simulink model "t_t_200_tge5"  (Simulink 6.2)
settings: Solver=ode45  StartTime=0.0  StopTime=10  RelTol=1e-3
undefined symbols (not defined in the file): BEE2_usr
libraries: xbsIndex_r3 x575, xps_library x48, casper_library x20
(part 3 of 4)

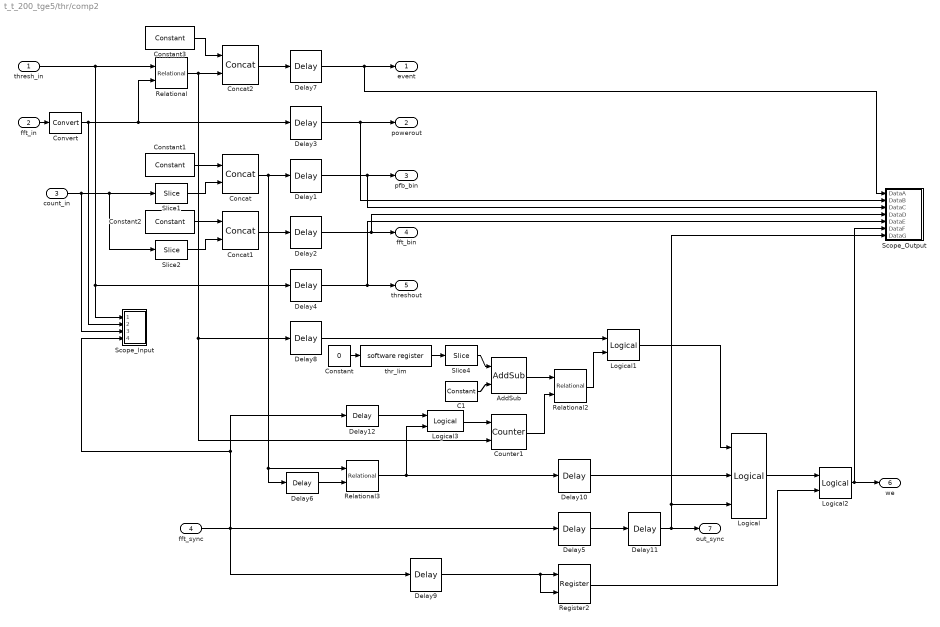
== system t_t_200_tge5/thr/comp2 ==
  thresh_in : Inport  Port=1  LatchInput=off
  fft_in : Inport  Port=2  LatchInput=off
  count_in : Inport  Port=3  LatchInput=off
  fft_sync : Inport  Port=4  LatchInput=off
  AddSub : xbsIndex_r3/AddSub  mode=Subtraction  precision=Full  arith_type=Unsigned  n_bits=8  bin_pt=2  quantization=Truncate  overflow=Wrap  latency=1  explicit_period=off  period=1  use_carryin=off  use_carryout=off  en=off  dbl_ovrd=off  show_param=off  use_core=on  pipeline=off  use_rpm=on  gen_core=off
      settings: xl_area=[0, 0, 0, 0, 0, 0, 0]
  C1 : xbsIndex_r3/Constant  const=1  equ=P=C  arith_type=Unsigned  n_bits=FFTSize  bin_pt=0  opselect=C  inp2=PCIN>>17  opr=+  inp1=P  carry=CIN  iostate=0  explicit_period=on  period=1  dbl_ovrd=off
  Concat : xbsIndex_r3/Concat  num_inputs=2  explicit_period=off  period=1  dbl_ovrd=off
  Concat1 : xbsIndex_r3/Concat  num_inputs=2  explicit_period=off  period=1  dbl_ovrd=off
  Concat2 : xbsIndex_r3/Concat  num_inputs=2  explicit_period=off  period=1  dbl_ovrd=off
  Constant : Constant  Value=0  OutDataTypeMode=double
  Constant1 : xbsIndex_r3/Constant  const=0  equ=P=C  arith_type=Unsigned  n_bits=CPUWidth - PFBSize  bin_pt=0  opselect=C  inp2=PCIN>>17  opr=+  inp1=P  carry=CIN  iostate=0  explicit_period=on  period=1  dbl_ovrd=off
  Constant2 : xbsIndex_r3/Constant  const=0  equ=P=C  arith_type=Unsigned  n_bits=CPUWidth - FFTSize  bin_pt=0  opselect=C  inp2=PCIN>>17  opr=+  inp1=P  carry=CIN  iostate=0  explicit_period=on  period=1  dbl_ovrd=off
  Constant3 : xbsIndex_r3/Constant  const=0  equ=P=C  arith_type=Unsigned  n_bits=CPUWidth-1  bin_pt=0  opselect=C  inp2=PCIN>>17  opr=+  inp1=P  carry=CIN  iostate=0  explicit_period=on  period=1  dbl_ovrd=off
  Convert : xbsIndex_r3/Convert  arith_type=Unsigned  n_bits=CPUWidth  bin_pt=CPUWidth - 3  quantization=Truncate  overflow=Wrap  latency=0  explicit_period=off  period=1  dbl_ovrd=off  show_param=off  inserted_by_tool=off  pipeline=off
      settings: xl_area=[0, 0, 0, 0, 0, 0, 0]
  Counter1 : xbsIndex_r3/Counter  cnt_type=Free Running  n_bits=FFTSize  bin_pt=0  arith_type=Unsigned  start_count=0  cnt_to=Inf  cnt_by_val=1  operation=Up  explicit_period=off  period=1  load_pin=off  rst=on  en=on  dbl_ovrd=off  show_param=off  use_rpm=on  gen_core=off
      settings: xl_area=[0, 0, 0, 0, 0, 0, 0]
  Delay{1..4} (4 alike) : xbsIndex_r3/Delay  latency=3  reg_retiming=on  explicit_period=off  period=1  en=off  accept_only_valid=off  init_zero=on  dbl_ovrd=off  show_param=off
      settings: xl_area=[0, 0, 0, 0, 0, 0, 0]
  Delay{6,8,10..12} (5 alike) : xbsIndex_r3/Delay  latency=1  reg_retiming=on  explicit_period=off  period=1  en=off  accept_only_valid=off  init_zero=on  dbl_ovrd=off  show_param=off
      settings: xl_area=[0, 0, 0, 0, 0, 0, 0]
  Delay5 : xbsIndex_r3/Delay  latency=2  reg_retiming=on  explicit_period=off  period=1  en=off  accept_only_valid=off  init_zero=on  dbl_ovrd=off  show_param=off
      settings: xl_area=[0, 0, 0, 0, 0, 0, 0]
  Delay7 : xbsIndex_r3/Delay  latency=2  reg_retiming=on  explicit_period=off  period=1  en=off  accept_only_valid=off  init_zero=on  dbl_ovrd=off  show_param=off
      settings: xl_area=[0, 0, 0, 0, 0, 0, 0]
  Delay9 : xbsIndex_r3/Delay  latency=2  reg_retiming=on  explicit_period=off  period=1  en=off  accept_only_valid=off  init_zero=on  dbl_ovrd=off  show_param=off
      settings: xl_area=[0, 0, 0, 0, 0, 0, 0]
  Logical : xbsIndex_r3/Logical  logical_function=OR  inputs=3  precision=Full  arith_type=Unsigned  n_bits=8  bin_pt=2  align_bp=on  latency=0  explicit_period=off  period=1  en=off  dbl_ovrd=off  show_param=off
      settings: xl_area=[0, 0, 0, 0, 0, 0, 0]
  Logical1 : xbsIndex_r3/Logical  logical_function=AND  inputs=2  precision=Full  arith_type=Unsigned  n_bits=8  bin_pt=2  align_bp=on  latency=0  explicit_period=off  period=1  en=off  dbl_ovrd=off  show_param=off
      settings: xl_area=[0, 0, 0, 0, 0, 0, 0]
  Logical2 : xbsIndex_r3/Logical  logical_function=AND  inputs=2  precision=Full  arith_type=Unsigned  n_bits=8  bin_pt=2  align_bp=on  latency=1  explicit_period=off  period=1  en=off  dbl_ovrd=off  show_param=off
      settings: xl_area=[0, 0, 0, 0, 0, 0, 0]
  Logical3 : xbsIndex_r3/Logical  logical_function=OR  inputs=2  precision=Full  arith_type=Unsigned  n_bits=8  bin_pt=2  align_bp=on  latency=0  explicit_period=off  period=1  en=off  dbl_ovrd=off  show_param=off
      settings: xl_area=[0, 0, 0, 0, 0, 0, 0]
  Register2 : xbsIndex_r3/Register  init=0  reg_only_valid=off  explicit_period=off  period=1  rst=off  en=on  out_en=off  dbl_ovrd=off  show_param=off
      settings: xl_area=[0, 0, 0, 0, 0, 0, 0]
  Relational : xbsIndex_r3/Relational  mode=a<b  latency=1  explicit_period=off  period=1  en=off  dbl_ovrd=off  show_param=off
      settings: xl_area=[0, 0, 0, 0, 0, 0, 0]
  Relational2 : xbsIndex_r3/Relational  mode=a>b  latency=1  explicit_period=off  period=1  en=off  dbl_ovrd=off  show_param=off
      settings: xl_area=[0, 0, 0, 0, 0, 0, 0]
  Relational3 : xbsIndex_r3/Relational  mode=a!=b  latency=1  explicit_period=off  period=1  en=off  dbl_ovrd=off  show_param=off
      settings: xl_area=[0, 0, 0, 0, 0, 0, 0]
  Scope_Input : Subsystem
  Scope_Output : Subsystem
  Slice1 : xbsIndex_r3/Slice  mode=Lower Bit Location + Width  nbits=PFBSize  bit1=0  base1=MSB of Input  bit0=FFTSize  base0=LSB of Input  boolean_output=off  explicit_period=off  period=1  dbl_ovrd=off
  Slice2 : xbsIndex_r3/Slice  mode=Lower Bit Location + Width  nbits=FFTSize  bit1=0  base1=MSB of Input  bit0=0  base0=LSB of Input  boolean_output=off  explicit_period=off  period=1  dbl_ovrd=off
  Slice4 : xbsIndex_r3/Slice  mode=Lower Bit Location + Width  nbits=FFTSize  bit1=0  base1=MSB of Input  bit0=0  base0=LSB of Input  boolean_output=off  explicit_period=off  period=1  dbl_ovrd=off
  thr_lim : xps_library/software register  Tag=xps:sw_reg  io_dir=From Processor  arith_type=Unsigned  bitwidth=32  bin_pt=0  sample_period=1  gw_name=t_t_200_tge5_thr_comp2_thr_lim_user_data_out
  event : Outport
  powerout : Outport  Port=2
  pfb_bin : Outport  Port=3
  fft_bin : Outport  Port=4
  threshout : Outport  Port=5
  we : Outport  Port=6
  out_sync : Outport  Port=7
  wires:
  thresh_in/1 -> Relational/1, Scope_Input/1(DataA), Delay4/1
  Relational/1 -> Delay8/1, Counter1/2, Concat2/2
  fft_in/1 -> Convert/1
  Delay3/1 -> powerout/1, Scope_Output/2(DataB)
  Slice2/1 -> Concat1/2
  Constant2/1 -> Concat1/1
  Slice1/1 -> Concat/2
  Constant1/1 -> Concat/1
  count_in/1 -> Slice1/1, Slice2/1, Scope_Input/3(DataC)
  Concat/1 -> Delay1/1, Relational3/1, Delay6/1
  Concat1/1 -> Delay2/1
  Delay1/1 -> pfb_bin/1, Scope_Output/3(DataC)
  Delay2/1 -> fft_bin/1, Scope_Output/4(DataD)
  Delay4/1 -> Scope_Output/5(DataE), threshout/1
  fft_sync/1 -> Scope_Input/4(Sync), Delay12/1, Delay5/1, Delay9/1
  Delay5/1 -> Delay11/1
  Constant/1 -> thr_lim/1
  thr_lim/1 -> Slice4/1
  Relational3/1 -> Delay10/1, Logical3/2
  Delay6/1 -> Relational3/2
  Relational2/1 -> Logical1/2
  Logical1/1 -> Logical/1
  Delay7/1 -> event/1, Scope_Output/1(DataA)
  Delay8/1 -> Logical1/1
  Slice4/1 -> AddSub/1
  C1/1 -> AddSub/2
  Counter1/1 -> Relational2/2
  AddSub/1 -> Relational2/1
  Delay10/1 -> Logical/2
  Concat2/1 -> Delay7/1
  Constant3/1 -> Concat2/1
  Logical3/1 -> Counter1/1
  Delay11/1 -> Scope_Output/7("DataG "), Logical/3, out_sync/1
  Logical/1 -> Logical2/1
  Logical2/1 -> we/1, Scope_Output/6("DataF ")
  Delay9/1 -> Register2/1, Register2/2
  Delay12/1 -> Logical3/1
  Register2/1 -> Logical2/2
  Convert/1 -> Delay3/1, Relational/2, Scope_Input/2(DataB)

== system t_t_200_tge5/thr/ct_power ==
  note: Reloaded 'c_to_ri' blocks.
      | May need to change
      | bitwidth and binary point
  din1 : Inport  Port=1  LatchInput=off
  din2 : Inport  Port=2  LatchInput=off
  din_sync : Inport  Port=3  LatchInput=off
  Scope_Input : Subsystem
  a1 : xbsIndex_r3/AddSub  mode=Addition  precision=Full  arith_type=Unsigned  n_bits=8  bin_pt=2  quantization=Truncate  overflow=Wrap  latency=add_lat  explicit_period=off  period=1  use_carryin=off  use_carryout=off  en=off  dbl_ovrd=off  show_param=off  use_core=on  pipeline=off  use_rpm=on  gen_core=off
      settings: xl_area=[0, 0, 0, 0, 0, 0, 0]
  a2 : xbsIndex_r3/AddSub  mode=Addition  precision=Full  arith_type=Unsigned  n_bits=8  bin_pt=2  quantization=Truncate  overflow=Wrap  latency=add_lat  explicit_period=off  period=1  use_carryin=off  use_carryout=off  en=off  dbl_ovrd=off  show_param=off  use_core=on  pipeline=off  use_rpm=on  gen_core=off
      settings: xl_area=[0, 0, 0, 0, 0, 0, 0]
  c_to_ri : casper_library/Misc/c_to_ri  n_bits=DataWidth  bin_pt=DataWidth - 1
      settings: AttributesFormatString=18_17 r/i
  c_to_ri1 : casper_library/Misc/c_to_ri  n_bits=DataWidth  bin_pt=DataWidth -1
      settings: AttributesFormatString=18_17 r/i
  delay_sync : xbsIndex_r3/Delay  latency=add_lat+mult_lat  reg_retiming=off  explicit_period=off  period=1  en=off  accept_only_valid=off  init_zero=on  dbl_ovrd=off  show_param=off
      settings: xl_area=[0, 0, 0, 0, 0, 0, 0]
  m{1..4} (4 alike) : xbsIndex_r3/Mult  precision=Full  arith_type=Unsigned  n_bits=2*DataWidth  bin_pt=2*(DataWidth-1)  quantization="Round  (unbiased: +/- Inf)"  overflow=Wrap  latency=mult_lat  explicit_period=on  period=-1  en=off  dbl_ovrd=off  show_param=on  mult_type=Parallel  oversample=2  use_embedded=on  pipeline=on  use_rpm=on  placement_style=Rectangular Shape  gen_core=off
      settings: xl_area=[0, 0, 0, 0, 0, 0, 0]
  pout1 : Outport
  pout2 : Outport  Port=2
  dout_sync : Outport  Port=3
  wires:
  din1/1 -> c_to_ri/1
  c_to_ri/1 -> Scope_Input/1(DataA), m1/1, m1/2
  c_to_ri/2 -> m2/2, m2/1, Scope_Input/2(DataB)
  din2/1 -> c_to_ri1/1
  c_to_ri1/1 -> m3/2, m3/1
  m2/1 -> Scope_Input/3(DataC), a1/2
  a1/1 -> Scope_Input/4(Sync), pout1/1
  m3/1 -> a2/1
  m4/1 -> a2/2
  a2/1 -> pout2/1
  m1/1 -> a1/1
  c_to_ri1/2 -> m4/1, m4/2
  delay_sync/1 -> dout_sync/1
  din_sync/1 -> delay_sync/1

== system t_t_200_tge5/thr/fft_power ==
  note: Reloaded 'c_to_ri' blocks.
      | May need to change
      | bitwidth and binary point
  din1 : Inport  Port=1  LatchInput=off
  din2 : Inport  Port=2  LatchInput=off
  din_sync : Inport  Port=3  LatchInput=off
  Scope_Input : Subsystem
  a1 : xbsIndex_r3/AddSub  mode=Addition  precision=Full  arith_type=Unsigned  n_bits=8  bin_pt=2  quantization=Truncate  overflow=Wrap  latency=add_lat  explicit_period=off  period=1  use_carryin=off  use_carryout=off  en=off  dbl_ovrd=off  show_param=off  use_core=on  pipeline=off  use_rpm=on  gen_core=off
      settings: xl_area=[0, 0, 0, 0, 0, 0, 0]
  a2 : xbsIndex_r3/AddSub  mode=Addition  precision=Full  arith_type=Unsigned  n_bits=8  bin_pt=2  quantization=Truncate  overflow=Wrap  latency=add_lat  explicit_period=off  period=1  use_carryin=off  use_carryout=off  en=off  dbl_ovrd=off  show_param=off  use_core=on  pipeline=off  use_rpm=on  gen_core=off
      settings: xl_area=[0, 0, 0, 0, 0, 0, 0]
  c_to_ri : casper_library/Misc/c_to_ri  n_bits=DataWidth  bin_pt=DataWidth-1
      settings: AttributesFormatString=18_17 r/i
  c_to_ri1 : casper_library/Misc/c_to_ri  n_bits=DataWidth  bin_pt=DataWidth - 1
      settings: AttributesFormatString=18_17 r/i
  delay_sync : xbsIndex_r3/Delay  latency=add_lat+mult_lat  reg_retiming=off  explicit_period=off  period=1  en=off  accept_only_valid=off  init_zero=on  dbl_ovrd=off  show_param=off
      settings: xl_area=[0, 0, 0, 0, 0, 0, 0]
  m{1..4} (4 alike) : xbsIndex_r3/Mult  precision=User Defined  arith_type=Unsigned  n_bits=2*DataWidth  bin_pt=2*(DataWidth-1)  quantization="Round  (unbiased: +/- Inf)"  overflow=Wrap  latency=mult_lat  explicit_period=on  period=-1  en=off  dbl_ovrd=off  show_param=on  mult_type=Parallel  oversample=2  use_embedded=on  pipeline=on  use_rpm=on  placement_style=Rectangular Shape  gen_core=off
      settings: xl_area=[0, 0, 0, 0, 0, 0, 0]
  pout1 : Outport
  pout2 : Outport  Port=2
  dout_sync : Outport  Port=3
  wires:
  din1/1 -> Scope_Input/3(DataC), c_to_ri/1
  c_to_ri/1 -> m1/1, m1/2
  c_to_ri/2 -> m2/1, m2/2
  din2/1 -> c_to_ri1/1
  c_to_ri1/1 -> m3/1, m3/2
  m2/1 -> a1/2
  a1/1 -> Scope_Input/1(DataA), pout1/1
  m3/1 -> a2/1
  m4/1 -> a2/2
  a2/1 -> Scope_Input/2(DataB), pout2/1
  m1/1 -> a1/1
  c_to_ri1/2 -> m4/2, m4/1
  delay_sync/1 -> Scope_Input/4(Sync), dout_sync/1
  din_sync/1 -> delay_sync/1

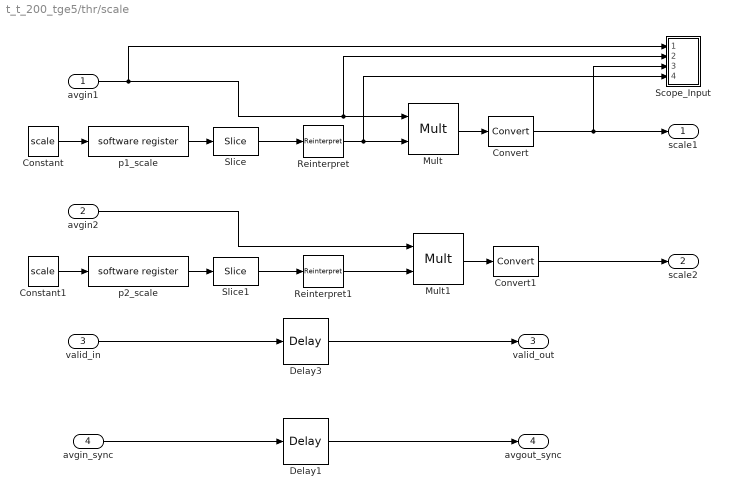
== system t_t_200_tge5/thr/scale ==
  avgin1 : Inport  Port=1  LatchInput=off
  avgin2 : Inport  Port=2  LatchInput=off
  valid_in : Inport  Port=3  LatchInput=off
  avgin_sync : Inport  Port=4  LatchInput=off
  Constant : Constant  Value=scale
  Constant1 : Constant  Value=scale
  Convert : xbsIndex_r3/Convert  arith_type=Unsigned  n_bits=2*DataWidth  bin_pt=2*DataWidth-2  quantization=Truncate  overflow=Wrap  latency=0  explicit_period=off  period=1  dbl_ovrd=off  show_param=off  inserted_by_tool=off  pipeline=off
      settings: xl_area=[0, 0, 0, 0, 0, 0, 0]
  Convert1 : xbsIndex_r3/Convert  arith_type=Unsigned  n_bits=2*DataWidth  bin_pt=2*DataWidth-2  quantization=Truncate  overflow=Wrap  latency=0  explicit_period=off  period=1  dbl_ovrd=off  show_param=off  inserted_by_tool=off  pipeline=off
      settings: xl_area=[0, 0, 0, 0, 0, 0, 0]
  Delay1 : xbsIndex_r3/Delay  latency=3  reg_retiming=off  explicit_period=off  period=1  en=off  accept_only_valid=off  init_zero=on  dbl_ovrd=off  show_param=off
      settings: xl_area=[0, 0, 0, 0, 0, 0, 0]
  Delay3 : xbsIndex_r3/Delay  latency=3  reg_retiming=off  explicit_period=off  period=1  en=off  accept_only_valid=off  init_zero=on  dbl_ovrd=off  show_param=off
      settings: xl_area=[0, 0, 0, 0, 0, 0, 0]
  Mult : xbsIndex_r3/Mult  precision=Full  arith_type="Signed  (2's comp)"  n_bits=8  bin_pt=2  quantization=Truncate  overflow=Wrap  latency=mult_lat  explicit_period=off  period=1  en=off  dbl_ovrd=off  show_param=on  mult_type=Parallel  oversample=2  use_embedded=on  pipeline=on  use_rpm=on  placement_style=Rectangular Shape  gen_core=off
      settings: xl_area=[0, 0, 0, 0, 0, 0, 0]
  Mult1 : xbsIndex_r3/Mult  precision=Full  arith_type="Signed  (2's comp)"  n_bits=8  bin_pt=2  quantization=Truncate  overflow=Wrap  latency=mult_lat  explicit_period=off  period=1  en=off  dbl_ovrd=off  show_param=on  mult_type=Parallel  oversample=2  use_embedded=on  pipeline=on  use_rpm=on  placement_style=Rectangular Shape  gen_core=off
      settings: xl_area=[0, 0, 0, 0, 0, 0, 0]
  Reinterpret : xbsIndex_r3/Reinterpret  force_arith_type=on  arith_type=Unsigned  force_bin_pt=on  bin_pt=DataWidth - ceil(DataWidth/2)  force_valid=on
  Reinterpret1 : xbsIndex_r3/Reinterpret  force_arith_type=on  arith_type=Unsigned  force_bin_pt=on  bin_pt=DataWidth - ceil(DataWidth/2)  force_valid=on
  Scope_Input : Subsystem
  Slice : xbsIndex_r3/Slice  mode=Lower Bit Location + Width  nbits=DataWidth  bit1=0  base1=LSB of Input  bit0=0  base0=LSB of Input  boolean_output=off  explicit_period=off  period=1  dbl_ovrd=off
  Slice1 : xbsIndex_r3/Slice  mode=Lower Bit Location + Width  nbits=DataWidth  bit1=0  base1=LSB of Input  bit0=0  base0=LSB of Input  boolean_output=off  explicit_period=off  period=1  dbl_ovrd=off
  p1_scale : xps_library/software register  Tag=xps:sw_reg  io_dir=From Processor  arith_type=Unsigned  bitwidth=32  bin_pt=ceil(DataWidth/2)  sample_period=1  gw_name=t_t_200_tge5_thr_scale_p1_scale_user_data_out
  p2_scale : xps_library/software register  Tag=xps:sw_reg  io_dir=From Processor  arith_type=Unsigned  bitwidth=32  bin_pt=ceil(DataWidth/2)  sample_period=1  gw_name=t_t_200_tge5_thr_scale_p2_scale_user_data_out
  scale1 : Outport
  scale2 : Outport  Port=2
  valid_out : Outport  Port=3
  avgout_sync : Outport  Port=4
  wires:
  Convert1/1 -> scale2/1
  Convert/1 -> Scope_Input/3(DataC), scale1/1
  avgin_sync/1 -> Delay1/1
  Delay1/1 -> avgout_sync/1
  Constant1/1 -> p2_scale/1
  Constant/1 -> p1_scale/1
  avgin2/1 -> Mult1/1
  Slice/1 -> Reinterpret/1
  Slice1/1 -> Reinterpret1/1
  p1_scale/1 -> Slice/1
  p2_scale/1 -> Slice1/1
  Reinterpret/1 -> Scope_Input/4(Sync), Mult/2
  avgin1/1 -> Scope_Input/2(DataB), Mult/1, Scope_Input/1(DataA)
  Reinterpret1/1 -> Mult1/2
  Mult/1 -> Convert/1
  Mult1/1 -> Convert1/1
  valid_in/1 -> Delay3/1
  Delay3/1 -> valid_out/1

== system t_t_200_tge5/ct_in_mux/tvg/bram_wr_out_sim ==
  Concat : xbsIndex_r3/Concat  num_inputs=5  explicit_period=off  period=1  dbl_ovrd=off
  Gateway Out : xbsIndex_r3/Gateway Out  output_type=Double  nbits=8  bin_pt=6  arith_type=Boolean  quantization=Truncate  overflow=Wrap  hdl_port=on  timing_constraint=None  locs_specified=off  LOCs={}  needs_fixed_name=off  show_param=off
      settings: xl_area=[0, 0, 0, 0, 0, 0, 0]
  RAM_sel : xbsIndex_r3/Constant  const=ram_sel  equ=P=C  arith_type=Unsigned  n_bits=2  bin_pt=0  opselect=C  inp2=PCIN>>17  opr=+  inp1=P  carry=CIN  iostate=0  explicit_period=on  period=1  dbl_ovrd=off
  WE : xbsIndex_r3/Constant  const=we_enable  equ=P=C  arith_type=Unsigned  n_bits=1  bin_pt=0  opselect=C  inp2=PCIN>>17  opr=+  inp1=P  carry=CIN  iostate=0  explicit_period=on  period=1  dbl_ovrd=off
  add_vec : xbsIndex_r3/Constant  const=add_vec  equ=P=C  arith_type=Unsigned  n_bits=9  bin_pt=0  opselect=C  inp2=PCIN>>17  opr=+  inp1=P  carry=CIN  iostate=0  explicit_period=on  period=1  dbl_ovrd=off
  data_in : xbsIndex_r3/Constant  const=data_in  equ=P=C  arith_type=Unsigned  n_bits=18  bin_pt=0  opselect=C  inp2=PCIN>>17  opr=+  inp1=P  carry=CIN  iostate=0  explicit_period=on  period=1  dbl_ovrd=off
  zeros : xbsIndex_r3/Constant  const=0  equ=P=C  arith_type=Unsigned  n_bits=2  bin_pt=0  opselect=C  inp2=PCIN>>17  opr=+  inp1=P  carry=CIN  iostate=0  explicit_period=on  period=1  dbl_ovrd=off
  Out1 : Outport
  wires:
  Gateway Out/1 -> Out1/1
  Concat/1 -> Gateway Out/1
  zeros/1 -> Concat/1
  WE/1 -> Concat/2
  RAM_sel/1 -> Concat/3
  add_vec/1 -> Concat/4
  data_in/1 -> Concat/5

== system t_t_200_tge5/ct_in_mux/tvg/thr_cpu_ctrl_sim ==
  Concat : xbsIndex_r3/Concat  num_inputs=4  explicit_period=off  period=1  dbl_ovrd=off
  Delay : xbsIndex_r3/Delay  latency=1  reg_retiming=off  explicit_period=off  period=1  en=off  accept_only_valid=off  init_zero=on  dbl_ovrd=off  show_param=off
      settings: xl_area=[0, 0, 0, 0, 0, 0, 0]
  Disregard Subsystem : xbsIndex_r3/Disregard Subsystem  Tag=discardX
      settings: AttributesFormatString=Disregard Subsystem\nFor Generation
  Gateway Out : xbsIndex_r3/Gateway Out  output_type=Double  nbits=8  bin_pt=6  arith_type=Boolean  quantization=Truncate  overflow=Wrap  hdl_port=off  timing_constraint=None  locs_specified=off  LOCs={}  needs_fixed_name=off  show_param=off
      settings: xl_area=[0, 0, 0, 0, 0, 0, 0]
  Length : xbsIndex_r3/Constant  const=tvg_length  equ=P=C  arith_type=Unsigned  n_bits=10  bin_pt=0  opselect=C  inp2=PCIN>>17  opr=+  inp1=P  carry=CIN  iostate=0  explicit_period=on  period=1  dbl_ovrd=off
  "Skip\t" : xbsIndex_r3/Constant  const=tvg_skip  equ=P=C  arith_type=Unsigned  n_bits=10  bin_pt=0  opselect=C  inp2=PCIN>>17  opr=+  inp1=P  carry=CIN  iostate=0  explicit_period=on  period=1  dbl_ovrd=off
  Stall : xbsIndex_r3/Constant  const=tvg_stall  equ=P=C  arith_type=Unsigned  n_bits=10  bin_pt=0  opselect=C  inp2=PCIN>>17  opr=+  inp1=P  carry=CIN  iostate=0  explicit_period=on  period=1  dbl_ovrd=off
  pad_zeroes : xbsIndex_r3/Constant  const=0  equ=P=C  arith_type=Unsigned  n_bits=2  bin_pt=0  opselect=C  inp2=PCIN>>17  opr=+  inp1=P  carry=CIN  iostate=0  explicit_period=on  period=1  dbl_ovrd=off
  out : Outport
  wires:
  "Skip\t"/1 -> Concat/4
  Delay/1 -> Gateway Out/1
  Concat/1 -> Delay/1
  Gateway Out/1 -> out/1
  Stall/1 -> Concat/3
  pad_zeroes/1 -> Concat/1
  Length/1 -> Concat/2

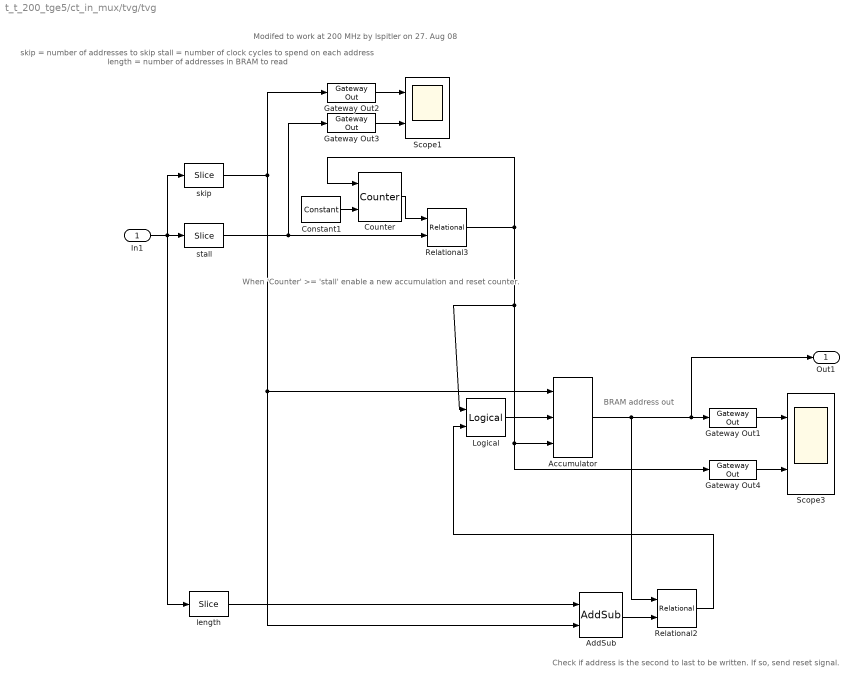
== system t_t_200_tge5/ct_in_mux/tvg/tvg ==
  note: Modifed to work at 200 MHz
      | by lspitler on 27. Aug 08
  note: BRAM address out
  note: Check if address is the
      | second to last to be written.
      | If so, send reset signal.
  note: When 'Counter' >= 'stall'
      | enable a new accumulation
      | and reset counter.
  note: skip = number of addresses to skip
      | stall = number of clock cycles to spend
      | on each address
      | length = number of addresses in BRAM
      | to read
  In1 : Inport  Port=1  LatchInput=off
  Accumulator : xbsIndex_r3/Accumulator  n_bits=10  overflow=Wrap  operation=Add  scale=1  explicit_period=on  period=1  rst=on  hasbypass=off  en=on  dbl_ovrd=off  show_param=off  gen_core=off  use_rpm=on
      settings: xl_area=[0, 0, 0, 0, 0, 0, 0]
  AddSub : xbsIndex_r3/AddSub  mode=Subtraction  precision=Full  arith_type=Unsigned  n_bits=8  bin_pt=2  quantization=Truncate  overflow=Wrap  latency=1  explicit_period=on  period=1  use_carryin=off  use_carryout=off  en=off  dbl_ovrd=off  show_param=off  use_core=on  pipeline=off  use_rpm=on  gen_core=off
      settings: xl_area=[0, 0, 0, 0, 0, 0, 0]
  Constant1 : xbsIndex_r3/Constant  const=1  equ=P=C  arith_type=Unsigned  n_bits=10  bin_pt=0  opselect=C  inp2=PCIN>>17  opr=+  inp1=P  carry=CIN  iostate=0  explicit_period=on  period=1  dbl_ovrd=off
  Counter : xbsIndex_r3/Counter  cnt_type=Free Running  n_bits=10  bin_pt=0  arith_type=Unsigned  start_count=0  cnt_to=inf  cnt_by_val=1  operation=Up  explicit_period=on  period=1  load_pin=on  rst=off  en=off  dbl_ovrd=off  show_param=off  use_rpm=on  gen_core=off
      settings: xl_area=[0, 0, 0, 0, 0, 0, 0]
  Gateway Out{1..4} (4 alike) : xbsIndex_r3/Gateway Out  output_type=Double  nbits=8  bin_pt=6  arith_type=Boolean  quantization=Truncate  overflow=Wrap  hdl_port=on  timing_constraint=None  locs_specified=off  LOCs={}  needs_fixed_name=off  show_param=off
      settings: xl_area=[0, 0, 0, 0, 0, 0, 0]
  Logical : xbsIndex_r3/Logical  logical_function=AND  inputs=2  precision=Full  arith_type=Unsigned  n_bits=8  bin_pt=2  align_bp=on  latency=0  explicit_period=off  period=1  en=off  dbl_ovrd=off  show_param=off
      settings: xl_area=[0, 0, 0, 0, 0, 0, 0]
  Relational2 : xbsIndex_r3/Relational  mode=a>=b  latency=0  explicit_period=on  period=1  en=off  dbl_ovrd=off  show_param=off
      settings: xl_area=[0, 0, 0, 0, 0, 0, 0]
  Relational3 : xbsIndex_r3/Relational  mode=a>=b  latency=0  explicit_period=on  period=1  en=off  dbl_ovrd=off  show_param=off
      settings: xl_area=[0, 0, 0, 0, 0, 0, 0]
  Scope1 : Scope  NumInputPorts=2
      settings: YMin=-5~-5  YMax=5~5
  Scope3 : Scope  NumInputPorts=2
      settings: TimeRange=20  YMin=-5~-5  YMax=5~5  SaveName=ScopeData4
  length : xbsIndex_r3/Slice  mode=Lower Bit Location + Width  nbits=10  bit1=0  base1=MSB of Input  bit0=20  base0=LSB of Input  boolean_output=off  explicit_period=on  period=1  dbl_ovrd=off
  skip : xbsIndex_r3/Slice  mode=Lower Bit Location + Width  nbits=10  bit1=0  base1=MSB of Input  bit0=0  base0=LSB of Input  boolean_output=off  explicit_period=on  period=1  dbl_ovrd=off
  stall : xbsIndex_r3/Slice  mode=Lower Bit Location + Width  nbits=10  bit1=0  base1=MSB of Input  bit0=10  base0=LSB of Input  boolean_output=off  explicit_period=on  period=1  dbl_ovrd=off
  Out1 : Outport
  wires:
  length/1 -> AddSub/1
  AddSub/1 -> Relational2/2
  In1/1 -> stall/1, skip/1, length/1
  Gateway Out1/1 -> Scope3/1
  Accumulator/1 -> Relational2/1, Out1/1, Gateway Out1/1
  skip/1 -> AddSub/2, Accumulator/1, Gateway Out2/1
  stall/1 -> Gateway Out3/1, Relational3/2
  Gateway Out2/1 -> Scope1/1
  Gateway Out3/1 -> Scope1/2
  Gateway Out4/1 -> Scope3/2
  Relational3/1 -> Counter/1, Accumulator/3, Gateway Out4/1, Logical/1
  Counter/1 -> Relational3/1
  Constant1/1 -> Counter/2
  Relational2/1 -> Logical/2
  Logical/1 -> Accumulator/2

== system t_t_200_tge5/fft_in_mux/tvg/bram_wr_out_sim ==
  Concat : xbsIndex_r3/Concat  num_inputs=5  explicit_period=off  period=1  dbl_ovrd=off
  Gateway Out : xbsIndex_r3/Gateway Out  output_type=Double  nbits=8  bin_pt=6  arith_type=Boolean  quantization=Truncate  overflow=Wrap  hdl_port=on  timing_constraint=None  locs_specified=off  LOCs={}  needs_fixed_name=off  show_param=off
      settings: xl_area=[0, 0, 0, 0, 0, 0, 0]
  RAM_sel : xbsIndex_r3/Constant  const=ram_sel  equ=P=C  arith_type=Unsigned  n_bits=2  bin_pt=0  opselect=C  inp2=PCIN>>17  opr=+  inp1=P  carry=CIN  iostate=0  explicit_period=on  period=1  dbl_ovrd=off
  WE : xbsIndex_r3/Constant  const=we_enable  equ=P=C  arith_type=Unsigned  n_bits=1  bin_pt=0  opselect=C  inp2=PCIN>>17  opr=+  inp1=P  carry=CIN  iostate=0  explicit_period=on  period=1  dbl_ovrd=off
  add_vec : xbsIndex_r3/Constant  const=add_vec  equ=P=C  arith_type=Unsigned  n_bits=9  bin_pt=0  opselect=C  inp2=PCIN>>17  opr=+  inp1=P  carry=CIN  iostate=0  explicit_period=on  period=1  dbl_ovrd=off
  data_in : xbsIndex_r3/Constant  const=data_in  equ=P=C  arith_type=Unsigned  n_bits=18  bin_pt=0  opselect=C  inp2=PCIN>>17  opr=+  inp1=P  carry=CIN  iostate=0  explicit_period=on  period=1  dbl_ovrd=off
  zeros : xbsIndex_r3/Constant  const=0  equ=P=C  arith_type=Unsigned  n_bits=2  bin_pt=0  opselect=C  inp2=PCIN>>17  opr=+  inp1=P  carry=CIN  iostate=0  explicit_period=on  period=1  dbl_ovrd=off
  Out1 : Outport
  wires:
  Gateway Out/1 -> Out1/1
  Concat/1 -> Gateway Out/1
  zeros/1 -> Concat/1
  WE/1 -> Concat/2
  RAM_sel/1 -> Concat/3
  add_vec/1 -> Concat/4
  data_in/1 -> Concat/5

== system t_t_200_tge5/fft_in_mux/tvg/thr_cpu_ctrl_sim ==
  Concat : xbsIndex_r3/Concat  num_inputs=4  explicit_period=off  period=1  dbl_ovrd=off
  Delay : xbsIndex_r3/Delay  latency=1  reg_retiming=off  explicit_period=off  period=1  en=off  accept_only_valid=off  init_zero=on  dbl_ovrd=off  show_param=off
      settings: xl_area=[0, 0, 0, 0, 0, 0, 0]
  Disregard Subsystem : xbsIndex_r3/Disregard Subsystem  Tag=discardX
      settings: AttributesFormatString=Disregard Subsystem\nFor Generation
  Gateway Out : xbsIndex_r3/Gateway Out  output_type=Double  nbits=8  bin_pt=6  arith_type=Boolean  quantization=Truncate  overflow=Wrap  hdl_port=off  timing_constraint=None  locs_specified=off  LOCs={}  needs_fixed_name=off  show_param=off
      settings: xl_area=[0, 0, 0, 0, 0, 0, 0]
  Length : xbsIndex_r3/Constant  const=tvg_length  equ=P=C  arith_type=Unsigned  n_bits=10  bin_pt=0  opselect=C  inp2=PCIN>>17  opr=+  inp1=P  carry=CIN  iostate=0  explicit_period=on  period=1  dbl_ovrd=off
  "Skip\t" : xbsIndex_r3/Constant  const=tvg_skip  equ=P=C  arith_type=Unsigned  n_bits=10  bin_pt=0  opselect=C  inp2=PCIN>>17  opr=+  inp1=P  carry=CIN  iostate=0  explicit_period=on  period=1  dbl_ovrd=off
  Stall : xbsIndex_r3/Constant  const=tvg_stall  equ=P=C  arith_type=Unsigned  n_bits=10  bin_pt=0  opselect=C  inp2=PCIN>>17  opr=+  inp1=P  carry=CIN  iostate=0  explicit_period=on  period=1  dbl_ovrd=off
  pad_zeroes : xbsIndex_r3/Constant  const=0  equ=P=C  arith_type=Unsigned  n_bits=2  bin_pt=0  opselect=C  inp2=PCIN>>17  opr=+  inp1=P  carry=CIN  iostate=0  explicit_period=on  period=1  dbl_ovrd=off
  out : Outport
  wires:
  "Skip\t"/1 -> Concat/4
  Delay/1 -> Gateway Out/1
  Concat/1 -> Delay/1
  Gateway Out/1 -> out/1
  Stall/1 -> Concat/3
  pad_zeroes/1 -> Concat/1
  Length/1 -> Concat/2

== system t_t_200_tge5/fft_in_mux/tvg/tvg ==
  note: Modifed to work at 200 MHz
      | by lspitler on 27. Aug 08
  note: BRAM address out
  note: Check if address is the
      | second to last to be written.
      | If so, send reset signal.
  note: When 'Counter' >= 'stall'
      | enable a new accumulation
      | and reset counter.
  note: skip = number of addresses to skip
      | stall = number of clock cycles to spend
      | on each address
      | length = number of addresses in BRAM
      | to read
  In1 : Inport  Port=1  LatchInput=off
  Accumulator : xbsIndex_r3/Accumulator  n_bits=10  overflow=Wrap  operation=Add  scale=1  explicit_period=on  period=1  rst=on  hasbypass=off  en=on  dbl_ovrd=off  show_param=off  gen_core=off  use_rpm=on
      settings: xl_area=[0, 0, 0, 0, 0, 0, 0]
  AddSub : xbsIndex_r3/AddSub  mode=Subtraction  precision=Full  arith_type=Unsigned  n_bits=8  bin_pt=2  quantization=Truncate  overflow=Wrap  latency=1  explicit_period=on  period=1  use_carryin=off  use_carryout=off  en=off  dbl_ovrd=off  show_param=off  use_core=on  pipeline=off  use_rpm=on  gen_core=off
      settings: xl_area=[0, 0, 0, 0, 0, 0, 0]
  Constant1 : xbsIndex_r3/Constant  const=1  equ=P=C  arith_type=Unsigned  n_bits=10  bin_pt=0  opselect=C  inp2=PCIN>>17  opr=+  inp1=P  carry=CIN  iostate=0  explicit_period=on  period=1  dbl_ovrd=off
  Counter : xbsIndex_r3/Counter  cnt_type=Free Running  n_bits=10  bin_pt=0  arith_type=Unsigned  start_count=0  cnt_to=inf  cnt_by_val=1  operation=Up  explicit_period=on  period=1  load_pin=on  rst=off  en=off  dbl_ovrd=off  show_param=off  use_rpm=on  gen_core=off
      settings: xl_area=[0, 0, 0, 0, 0, 0, 0]
  Gateway Out{1..4} (4 alike) : xbsIndex_r3/Gateway Out  output_type=Double  nbits=8  bin_pt=6  arith_type=Boolean  quantization=Truncate  overflow=Wrap  hdl_port=on  timing_constraint=None  locs_specified=off  LOCs={}  needs_fixed_name=off  show_param=off
      settings: xl_area=[0, 0, 0, 0, 0, 0, 0]
  Logical : xbsIndex_r3/Logical  logical_function=AND  inputs=2  precision=Full  arith_type=Unsigned  n_bits=8  bin_pt=2  align_bp=on  latency=0  explicit_period=off  period=1  en=off  dbl_ovrd=off  show_param=off
      settings: xl_area=[0, 0, 0, 0, 0, 0, 0]
  Relational2 : xbsIndex_r3/Relational  mode=a>=b  latency=0  explicit_period=on  period=1  en=off  dbl_ovrd=off  show_param=off
      settings: xl_area=[0, 0, 0, 0, 0, 0, 0]
  Relational3 : xbsIndex_r3/Relational  mode=a>=b  latency=0  explicit_period=on  period=1  en=off  dbl_ovrd=off  show_param=off
      settings: xl_area=[0, 0, 0, 0, 0, 0, 0]
  Scope1 : Scope  NumInputPorts=2
      settings: YMin=-5~-5  YMax=5~5
  Scope3 : Scope  NumInputPorts=2
      settings: TimeRange=20  YMin=-5~-5  YMax=5~5  SaveName=ScopeData4
  length : xbsIndex_r3/Slice  mode=Lower Bit Location + Width  nbits=10  bit1=0  base1=MSB of Input  bit0=20  base0=LSB of Input  boolean_output=off  explicit_period=on  period=1  dbl_ovrd=off
  skip : xbsIndex_r3/Slice  mode=Lower Bit Location + Width  nbits=10  bit1=0  base1=MSB of Input  bit0=0  base0=LSB of Input  boolean_output=off  explicit_period=on  period=1  dbl_ovrd=off
  stall : xbsIndex_r3/Slice  mode=Lower Bit Location + Width  nbits=10  bit1=0  base1=MSB of Input  bit0=10  base0=LSB of Input  boolean_output=off  explicit_period=on  period=1  dbl_ovrd=off
  Out1 : Outport
  wires:
  length/1 -> AddSub/1
  AddSub/1 -> Relational2/2
  In1/1 -> stall/1, skip/1, length/1
  Gateway Out1/1 -> Scope3/1
  Accumulator/1 -> Relational2/1, Out1/1, Gateway Out1/1
  skip/1 -> AddSub/2, Accumulator/1, Gateway Out2/1
  stall/1 -> Gateway Out3/1, Relational3/2
  Gateway Out2/1 -> Scope1/1
  Gateway Out3/1 -> Scope1/2
  Gateway Out4/1 -> Scope3/2
  Relational3/1 -> Counter/1, Accumulator/3, Gateway Out4/1, Logical/1
  Counter/1 -> Relational3/1
  Constant1/1 -> Counter/2
  Relational2/1 -> Logical/2
  Logical/1 -> Accumulator/2

== system t_t_200_tge5/thr/avg/Scope_Input ==
  DataA : Inport  Port=1  LatchInput=off
  DataB : Inport  Port=2  LatchInput=off
  DataC : Inport  Port=3  LatchInput=off
  Sync : Inport  Port=4  LatchInput=off
  Gateway Out{1..4} (4 alike) : xbsIndex_r3/Gateway Out  output_type=Double  nbits=8  bin_pt=6  arith_type=Boolean  quantization=Truncate  overflow=Wrap  hdl_port=off  timing_constraint=None  locs_specified=off  LOCs={}  needs_fixed_name=off  show_param=off
      settings: xl_area=[0, 0, 0, 0, 0, 0, 0]
  scope_ct_p1 : Scope  NumInputPorts=4
      settings: TimeRange=225.9933774834437  YMin=0~0~0~0  YMax=0.014~0.02~140~1
  wires:
  Sync/1 -> Gateway Out4/1
  Gateway Out4/1 -> scope_ct_p1/4
  DataC/1 -> Gateway Out3/1
  Gateway Out3/1 -> scope_ct_p1/3
  DataA/1 -> Gateway Out2/1
  Gateway Out1/1 -> scope_ct_p1/2
  DataB/1 -> Gateway Out1/1
  Gateway Out2/1 -> scope_ct_p1/1

== system t_t_200_tge5/thr/comp1/in_fft ==
  din : Inport  Port=1  LatchInput=off
  trig : Inport  Port=2  LatchInput=off
  en : Inport  Port=3  LatchInput=off
  Constant5 : xbsIndex_r3/Constant  const=1  equ=P=C  arith_type=Boolean  n_bits=1  bin_pt=0  opselect=C  inp2=PCIN>>17  opr=+  inp1=P  carry=CIN  iostate=0  explicit_period=on  period=1  dbl_ovrd=off
  Gateway Out : xbsIndex_r3/Gateway Out  output_type=Double  nbits=8  bin_pt=6  arith_type=Boolean  quantization=Truncate  overflow=Wrap  hdl_port=off  timing_constraint=None  locs_specified=off  LOCs={}  needs_fixed_name=off  show_param=off
      settings: xl_area=[0, 0, 0, 0, 0, 0, 0]
  Gateway Out1 : xbsIndex_r3/Gateway Out  output_type=Double  nbits=8  bin_pt=6  arith_type=Boolean  quantization=Truncate  overflow=Wrap  hdl_port=off  timing_constraint=None  locs_specified=off  LOCs={}  needs_fixed_name=off  show_param=off
      settings: xl_area=[0, 0, 0, 0, 0, 0, 0]
  Logical : xbsIndex_r3/Logical  logical_function=AND  inputs=2  precision=Full  arith_type=Unsigned  n_bits=8  bin_pt=2  align_bp=on  latency=0  explicit_period=on  period=1  en=off  dbl_ovrd=off  show_param=off
      settings: xl_area=[0, 0, 0, 0, 0, 0, 0]
  Reinterpret : xbsIndex_r3/Reinterpret  force_arith_type=on  arith_type=Unsigned  force_bin_pt=on  bin_pt=0  force_valid=on
  Scope : Scope  NumInputPorts=2
      settings: YMin=-5~-5  YMax=5~5
  bram : xps_library/Shared BRAM  Tag=xps:bram  arith_type=Unsigned  addr_width=nsamples  data_width=32  data_bin_pt=0  init_vals=zeros(1,4096)  sample_rate=1
  freeze_cntr : Subsystem  mask{CounterBits=nsamples}
      mask prompts: CounterBits "Counter Length (2^?)"
  posedge : Subsystem  Tag=Rising Edge Detector
  wires:
  Gateway Out1/1 -> Scope/2
  Gateway Out/1 -> Scope/1
  bram/1 -> Gateway Out/1
  freeze_cntr/1(addr) -> bram/1
  en/1 -> Logical/1
  trig/1 -> Logical/2
  posedge/1(Out) -> freeze_cntr/2(rst)
  Logical/1 -> posedge/1(In)
  freeze_cntr/2(we) -> Gateway Out1/1, bram/3
  Constant5/1 -> freeze_cntr/1(en)
  Reinterpret/1 -> bram/2
  din/1 -> Reinterpret/1

== system t_t_200_tge5/thr/comp1/in_thr ==
  din : Inport  Port=1  LatchInput=off
  trig : Inport  Port=2  LatchInput=off
  en : Inport  Port=3  LatchInput=off
  Constant5 : xbsIndex_r3/Constant  const=1  equ=P=C  arith_type=Boolean  n_bits=1  bin_pt=0  opselect=C  inp2=PCIN>>17  opr=+  inp1=P  carry=CIN  iostate=0  explicit_period=on  period=1  dbl_ovrd=off
  Gateway Out : xbsIndex_r3/Gateway Out  output_type=Double  nbits=8  bin_pt=6  arith_type=Boolean  quantization=Truncate  overflow=Wrap  hdl_port=off  timing_constraint=None  locs_specified=off  LOCs={}  needs_fixed_name=off  show_param=off
      settings: xl_area=[0, 0, 0, 0, 0, 0, 0]
  Gateway Out1 : xbsIndex_r3/Gateway Out  output_type=Double  nbits=8  bin_pt=6  arith_type=Boolean  quantization=Truncate  overflow=Wrap  hdl_port=off  timing_constraint=None  locs_specified=off  LOCs={}  needs_fixed_name=off  show_param=off
      settings: xl_area=[0, 0, 0, 0, 0, 0, 0]
  Logical : xbsIndex_r3/Logical  logical_function=AND  inputs=2  precision=Full  arith_type=Unsigned  n_bits=8  bin_pt=2  align_bp=on  latency=0  explicit_period=on  period=1  en=off  dbl_ovrd=off  show_param=off
      settings: xl_area=[0, 0, 0, 0, 0, 0, 0]
  Reinterpret : xbsIndex_r3/Reinterpret  force_arith_type=on  arith_type=Unsigned  force_bin_pt=on  bin_pt=0  force_valid=on
  Scope : Scope  NumInputPorts=2
      settings: YMin=-5~-5  YMax=5~5
  bram : xps_library/Shared BRAM  Tag=xps:bram  arith_type=Unsigned  addr_width=nsamples  data_width=32  data_bin_pt=0  init_vals=zeros(1,4096)  sample_rate=1
  freeze_cntr : Subsystem  mask{CounterBits=nsamples}
      mask prompts: CounterBits "Counter Length (2^?)"
  posedge : Subsystem  Tag=Rising Edge Detector
  wires:
  din/1 -> Reinterpret/1
  Reinterpret/1 -> bram/2
  Constant5/1 -> freeze_cntr/1(en)
  freeze_cntr/2(we) -> bram/3, Gateway Out1/1
  Logical/1 -> posedge/1(In)
  posedge/1(Out) -> freeze_cntr/2(rst)
  trig/1 -> Logical/2
  en/1 -> Logical/1
  freeze_cntr/1(addr) -> bram/1
  bram/1 -> Gateway Out/1
  Gateway Out/1 -> Scope/1
  Gateway Out1/1 -> Scope/2

== system t_t_200_tge5/thr/comp1/out_event ==
  din : Inport  Port=1  LatchInput=off
  trig : Inport  Port=2  LatchInput=off
  en : Inport  Port=3  LatchInput=off
  Constant5 : xbsIndex_r3/Constant  const=1  equ=P=C  arith_type=Boolean  n_bits=1  bin_pt=0  opselect=C  inp2=PCIN>>17  opr=+  inp1=P  carry=CIN  iostate=0  explicit_period=on  period=1  dbl_ovrd=off
  Gateway Out : xbsIndex_r3/Gateway Out  output_type=Double  nbits=8  bin_pt=6  arith_type=Boolean  quantization=Truncate  overflow=Wrap  hdl_port=off  timing_constraint=None  locs_specified=off  LOCs={}  needs_fixed_name=off  show_param=off
      settings: xl_area=[0, 0, 0, 0, 0, 0, 0]
  Gateway Out1 : xbsIndex_r3/Gateway Out  output_type=Double  nbits=8  bin_pt=6  arith_type=Boolean  quantization=Truncate  overflow=Wrap  hdl_port=off  timing_constraint=None  locs_specified=off  LOCs={}  needs_fixed_name=off  show_param=off
      settings: xl_area=[0, 0, 0, 0, 0, 0, 0]
  Logical : xbsIndex_r3/Logical  logical_function=AND  inputs=2  precision=Full  arith_type=Unsigned  n_bits=8  bin_pt=2  align_bp=on  latency=0  explicit_period=on  period=1  en=off  dbl_ovrd=off  show_param=off
      settings: xl_area=[0, 0, 0, 0, 0, 0, 0]
  Reinterpret : xbsIndex_r3/Reinterpret  force_arith_type=on  arith_type=Unsigned  force_bin_pt=on  bin_pt=0  force_valid=on
  Scope : Scope  NumInputPorts=2
      settings: YMin=-5~-5  YMax=5~5
  bram : xps_library/Shared BRAM  Tag=xps:bram  arith_type=Unsigned  addr_width=nsamples  data_width=32  data_bin_pt=0  init_vals=zeros(1,4096)  sample_rate=1
  freeze_cntr : Subsystem  mask{CounterBits=nsamples}
      mask prompts: CounterBits "Counter Length (2^?)"
  posedge : Subsystem  Tag=Rising Edge Detector
  wires:
  din/1 -> Reinterpret/1
  Reinterpret/1 -> bram/2
  Constant5/1 -> freeze_cntr/1(en)
  freeze_cntr/2(we) -> bram/3, Gateway Out1/1
  Logical/1 -> posedge/1(In)
  posedge/1(Out) -> freeze_cntr/2(rst)
  trig/1 -> Logical/2
  en/1 -> Logical/1
  freeze_cntr/1(addr) -> bram/1
  bram/1 -> Gateway Out/1
  Gateway Out/1 -> Scope/1
  Gateway Out1/1 -> Scope/2

== system t_t_200_tge5/thr/comp1/out_fft ==
  din : Inport  Port=1  LatchInput=off
  trig : Inport  Port=2  LatchInput=off
  en : Inport  Port=3  LatchInput=off
  Constant5 : xbsIndex_r3/Constant  const=1  equ=P=C  arith_type=Boolean  n_bits=1  bin_pt=0  opselect=C  inp2=PCIN>>17  opr=+  inp1=P  carry=CIN  iostate=0  explicit_period=on  period=1  dbl_ovrd=off
  Gateway Out : xbsIndex_r3/Gateway Out  output_type=Double  nbits=8  bin_pt=6  arith_type=Boolean  quantization=Truncate  overflow=Wrap  hdl_port=off  timing_constraint=None  locs_specified=off  LOCs={}  needs_fixed_name=off  show_param=off
      settings: xl_area=[0, 0, 0, 0, 0, 0, 0]
  Gateway Out1 : xbsIndex_r3/Gateway Out  output_type=Double  nbits=8  bin_pt=6  arith_type=Boolean  quantization=Truncate  overflow=Wrap  hdl_port=off  timing_constraint=None  locs_specified=off  LOCs={}  needs_fixed_name=off  show_param=off
      settings: xl_area=[0, 0, 0, 0, 0, 0, 0]
  Logical : xbsIndex_r3/Logical  logical_function=AND  inputs=2  precision=Full  arith_type=Unsigned  n_bits=8  bin_pt=2  align_bp=on  latency=0  explicit_period=on  period=1  en=off  dbl_ovrd=off  show_param=off
      settings: xl_area=[0, 0, 0, 0, 0, 0, 0]
  Reinterpret : xbsIndex_r3/Reinterpret  force_arith_type=on  arith_type=Unsigned  force_bin_pt=on  bin_pt=0  force_valid=on
  Scope : Scope  NumInputPorts=2
      settings: YMin=-5~-5  YMax=5~5
  bram : xps_library/Shared BRAM  Tag=xps:bram  arith_type=Unsigned  addr_width=nsamples  data_width=32  data_bin_pt=0  init_vals=zeros(1,4096)  sample_rate=1
  freeze_cntr : Subsystem  mask{CounterBits=nsamples}
      mask prompts: CounterBits "Counter Length (2^?)"
  posedge : Subsystem  Tag=Rising Edge Detector
  wires:
  Gateway Out1/1 -> Scope/2
  Gateway Out/1 -> Scope/1
  bram/1 -> Gateway Out/1
  freeze_cntr/1(addr) -> bram/1
  en/1 -> Logical/1
  trig/1 -> Logical/2
  posedge/1(Out) -> freeze_cntr/2(rst)
  Logical/1 -> posedge/1(In)
  freeze_cntr/2(we) -> Gateway Out1/1, bram/3
  Constant5/1 -> freeze_cntr/1(en)
  Reinterpret/1 -> bram/2
  din/1 -> Reinterpret/1

== system t_t_200_tge5/thr/comp1/out_pfb ==
  din : Inport  Port=1  LatchInput=off
  trig : Inport  Port=2  LatchInput=off
  en : Inport  Port=3  LatchInput=off
  Constant5 : xbsIndex_r3/Constant  const=1  equ=P=C  arith_type=Boolean  n_bits=1  bin_pt=0  opselect=C  inp2=PCIN>>17  opr=+  inp1=P  carry=CIN  iostate=0  explicit_period=on  period=1  dbl_ovrd=off
  Gateway Out : xbsIndex_r3/Gateway Out  output_type=Double  nbits=8  bin_pt=6  arith_type=Boolean  quantization=Truncate  overflow=Wrap  hdl_port=off  timing_constraint=None  locs_specified=off  LOCs={}  needs_fixed_name=off  show_param=off
      settings: xl_area=[0, 0, 0, 0, 0, 0, 0]
  Gateway Out1 : xbsIndex_r3/Gateway Out  output_type=Double  nbits=8  bin_pt=6  arith_type=Boolean  quantization=Truncate  overflow=Wrap  hdl_port=off  timing_constraint=None  locs_specified=off  LOCs={}  needs_fixed_name=off  show_param=off
      settings: xl_area=[0, 0, 0, 0, 0, 0, 0]
  Logical : xbsIndex_r3/Logical  logical_function=AND  inputs=2  precision=Full  arith_type=Unsigned  n_bits=8  bin_pt=2  align_bp=on  latency=0  explicit_period=on  period=1  en=off  dbl_ovrd=off  show_param=off
      settings: xl_area=[0, 0, 0, 0, 0, 0, 0]
  Reinterpret : xbsIndex_r3/Reinterpret  force_arith_type=on  arith_type=Unsigned  force_bin_pt=on  bin_pt=0  force_valid=on
  Scope : Scope  NumInputPorts=2
      settings: YMin=-5~-5  YMax=5~5
  bram : xps_library/Shared BRAM  Tag=xps:bram  arith_type=Unsigned  addr_width=nsamples  data_width=32  data_bin_pt=0  init_vals=zeros(1,4096)  sample_rate=1
  freeze_cntr : Subsystem  mask{CounterBits=nsamples}
      mask prompts: CounterBits "Counter Length (2^?)"
  posedge : Subsystem  Tag=Rising Edge Detector
  wires:
  din/1 -> Reinterpret/1
  Reinterpret/1 -> bram/2
  Constant5/1 -> freeze_cntr/1(en)
  freeze_cntr/2(we) -> bram/3, Gateway Out1/1
  Logical/1 -> posedge/1(In)
  posedge/1(Out) -> freeze_cntr/2(rst)
  trig/1 -> Logical/2
  en/1 -> Logical/1
  freeze_cntr/1(addr) -> bram/1
  bram/1 -> Gateway Out/1
  Gateway Out/1 -> Scope/1
  Gateway Out1/1 -> Scope/2

== system t_t_200_tge5/thr/comp1/out_pwr ==
  din : Inport  Port=1  LatchInput=off
  trig : Inport  Port=2  LatchInput=off
  en : Inport  Port=3  LatchInput=off
  Constant5 : xbsIndex_r3/Constant  const=1  equ=P=C  arith_type=Boolean  n_bits=1  bin_pt=0  opselect=C  inp2=PCIN>>17  opr=+  inp1=P  carry=CIN  iostate=0  explicit_period=on  period=1  dbl_ovrd=off
  Gateway Out : xbsIndex_r3/Gateway Out  output_type=Double  nbits=8  bin_pt=6  arith_type=Boolean  quantization=Truncate  overflow=Wrap  hdl_port=off  timing_constraint=None  locs_specified=off  LOCs={}  needs_fixed_name=off  show_param=off
      settings: xl_area=[0, 0, 0, 0, 0, 0, 0]
  Gateway Out1 : xbsIndex_r3/Gateway Out  output_type=Double  nbits=8  bin_pt=6  arith_type=Boolean  quantization=Truncate  overflow=Wrap  hdl_port=off  timing_constraint=None  locs_specified=off  LOCs={}  needs_fixed_name=off  show_param=off
      settings: xl_area=[0, 0, 0, 0, 0, 0, 0]
  Logical : xbsIndex_r3/Logical  logical_function=AND  inputs=2  precision=Full  arith_type=Unsigned  n_bits=8  bin_pt=2  align_bp=on  latency=0  explicit_period=on  period=1  en=off  dbl_ovrd=off  show_param=off
      settings: xl_area=[0, 0, 0, 0, 0, 0, 0]
  Reinterpret : xbsIndex_r3/Reinterpret  force_arith_type=on  arith_type=Unsigned  force_bin_pt=on  bin_pt=0  force_valid=on
  Scope : Scope  NumInputPorts=2
      settings: YMin=-5~-5  YMax=5~5
  bram : xps_library/Shared BRAM  Tag=xps:bram  arith_type=Unsigned  addr_width=nsamples  data_width=32  data_bin_pt=0  init_vals=zeros(1,4096)  sample_rate=1
  freeze_cntr : Subsystem  mask{CounterBits=nsamples}
      mask prompts: CounterBits "Counter Length (2^?)"
  posedge : Subsystem  Tag=Rising Edge Detector
  wires:
  Gateway Out1/1 -> Scope/2
  Gateway Out/1 -> Scope/1
  bram/1 -> Gateway Out/1
  freeze_cntr/1(addr) -> bram/1
  en/1 -> Logical/1
  trig/1 -> Logical/2
  posedge/1(Out) -> freeze_cntr/2(rst)
  Logical/1 -> posedge/1(In)
  freeze_cntr/2(we) -> Gateway Out1/1, bram/3
  Constant5/1 -> freeze_cntr/1(en)
  Reinterpret/1 -> bram/2
  din/1 -> Reinterpret/1

== system t_t_200_tge5/thr/comp1/out_thr ==
  din : Inport  Port=1  LatchInput=off
  trig : Inport  Port=2  LatchInput=off
  en : Inport  Port=3  LatchInput=off
  Constant5 : xbsIndex_r3/Constant  const=1  equ=P=C  arith_type=Boolean  n_bits=1  bin_pt=0  opselect=C  inp2=PCIN>>17  opr=+  inp1=P  carry=CIN  iostate=0  explicit_period=on  period=1  dbl_ovrd=off
  Gateway Out : xbsIndex_r3/Gateway Out  output_type=Double  nbits=8  bin_pt=6  arith_type=Boolean  quantization=Truncate  overflow=Wrap  hdl_port=off  timing_constraint=None  locs_specified=off  LOCs={}  needs_fixed_name=off  show_param=off
      settings: xl_area=[0, 0, 0, 0, 0, 0, 0]
  Gateway Out1 : xbsIndex_r3/Gateway Out  output_type=Double  nbits=8  bin_pt=6  arith_type=Boolean  quantization=Truncate  overflow=Wrap  hdl_port=off  timing_constraint=None  locs_specified=off  LOCs={}  needs_fixed_name=off  show_param=off
      settings: xl_area=[0, 0, 0, 0, 0, 0, 0]
  Logical : xbsIndex_r3/Logical  logical_function=AND  inputs=2  precision=Full  arith_type=Unsigned  n_bits=8  bin_pt=2  align_bp=on  latency=1  explicit_period=on  period=1  en=off  dbl_ovrd=off  show_param=off
      settings: xl_area=[0, 0, 0, 0, 0, 0, 0]
  Reinterpret : xbsIndex_r3/Reinterpret  force_arith_type=on  arith_type=Unsigned  force_bin_pt=on  bin_pt=0  force_valid=on
  Scope : Scope  NumInputPorts=2
      settings: YMin=-5~-5  YMax=5~5
  bram : xps_library/Shared BRAM  Tag=xps:bram  arith_type=Unsigned  addr_width=nsamples  data_width=32  data_bin_pt=0  init_vals=zeros(1,4096)  sample_rate=1
  freeze_cntr : Subsystem  mask{CounterBits=nsamples}
      mask prompts: CounterBits "Counter Length (2^?)"
  posedge : Subsystem  Tag=Rising Edge Detector
  wires:
  din/1 -> Reinterpret/1
  Reinterpret/1 -> bram/2
  Constant5/1 -> freeze_cntr/1(en)
  freeze_cntr/2(we) -> bram/3, Gateway Out1/1
  Logical/1 -> posedge/1(In)
  posedge/1(Out) -> freeze_cntr/2(rst)
  trig/1 -> Logical/2
  en/1 -> Logical/1
  freeze_cntr/1(addr) -> bram/1
  bram/1 -> Gateway Out/1
  Gateway Out/1 -> Scope/1
  Gateway Out1/1 -> Scope/2

== system t_t_200_tge5/thr/comp2/Scope_Input ==
  DataA : Inport  Port=1  LatchInput=off
  DataB : Inport  Port=2  LatchInput=off
  DataC : Inport  Port=3  LatchInput=off
  Sync : Inport  Port=4  LatchInput=off
  Gateway Out{1..4} (4 alike) : xbsIndex_r3/Gateway Out  output_type=Double  nbits=8  bin_pt=6  arith_type=Boolean  quantization=Truncate  overflow=Wrap  hdl_port=off  timing_constraint=None  locs_specified=off  LOCs={}  needs_fixed_name=off  show_param=off
      settings: xl_area=[0, 0, 0, 0, 0, 0, 0]
  scope_ct_p1 : Scope  NumInputPorts=4
      settings: TimeRange=225.9933774834437  YMin=0~0~0~0  YMax=0.014~0.02~140~1
  wires:
  Gateway Out2/1 -> scope_ct_p1/1
  DataB/1 -> Gateway Out1/1
  Gateway Out1/1 -> scope_ct_p1/2
  DataA/1 -> Gateway Out2/1
  Gateway Out3/1 -> scope_ct_p1/3
  DataC/1 -> Gateway Out3/1
  Gateway Out4/1 -> scope_ct_p1/4
  Sync/1 -> Gateway Out4/1

== system t_t_200_tge5/thr/comp2/Scope_Output ==
  DataA : Inport  Port=1  LatchInput=off
  DataB : Inport  Port=2  LatchInput=off
  DataC : Inport  Port=3  LatchInput=off
  DataD : Inport  Port=4  LatchInput=off
  DataE : Inport  Port=5  LatchInput=off
  "DataF " : Inport  Port=6  LatchInput=off
  "DataG " : Inport  Port=7  LatchInput=off
  Gateway Out{1..7} (7 alike) : xbsIndex_r3/Gateway Out  output_type=Double  nbits=8  bin_pt=6  arith_type=Boolean  quantization=Truncate  overflow=Wrap  hdl_port=off  timing_constraint=None  locs_specified=off  LOCs={}  needs_fixed_name=off  show_param=off
      settings: xl_area=[0, 0, 0, 0, 0, 0, 0]
  Scope_output : Scope  NumInputPorts=7
      settings: TimeRange=152.1280625333588  YMin=0~0~0~0~0~0~0  YMax=1~0.01~40~150~0.01~1~1
  wires:
  DataD/1 -> Gateway Out4/1
  DataC/1 -> Gateway Out3/1
  DataA/1 -> Gateway Out2/1
  DataB/1 -> Gateway Out1/1
  DataE/1 -> Gateway Out5/1
  "DataF "/1 -> Gateway Out6/1
  "DataG "/1 -> Gateway Out7/1
  Gateway Out4/1 -> Scope_output/4
  Gateway Out3/1 -> Scope_output/3
  Gateway Out1/1 -> Scope_output/2
  Gateway Out2/1 -> Scope_output/1
  Gateway Out5/1 -> Scope_output/5
  Gateway Out6/1 -> Scope_output/6
  Gateway Out7/1 -> Scope_output/7

== system t_t_200_tge5/thr/ct_power/Scope_Input ==
  DataA : Inport  Port=1  LatchInput=off
  DataB : Inport  Port=2  LatchInput=off
  DataC : Inport  Port=3  LatchInput=off
  Sync : Inport  Port=4  LatchInput=off
  Gateway Out{1..4} (4 alike) : xbsIndex_r3/Gateway Out  output_type=Double  nbits=8  bin_pt=6  arith_type=Boolean  quantization=Truncate  overflow=Wrap  hdl_port=off  timing_constraint=None  locs_specified=off  LOCs={}  needs_fixed_name=off  show_param=off
      settings: xl_area=[0, 0, 0, 0, 0, 0, 0]
  scope_ct_p1 : Scope  NumInputPorts=4
      settings: TimeRange=225.9933774834437  YMin=0~0~0~0  YMax=0.014~0.02~140~1
  wires:
  Sync/1 -> Gateway Out4/1
  Gateway Out4/1 -> scope_ct_p1/4
  DataC/1 -> Gateway Out3/1
  Gateway Out3/1 -> scope_ct_p1/3
  DataA/1 -> Gateway Out2/1
  Gateway Out1/1 -> scope_ct_p1/2
  DataB/1 -> Gateway Out1/1
  Gateway Out2/1 -> scope_ct_p1/1
